simulink model "Eg8_4"  (R2018a)
settings: Solver=VariableStepAuto  StartTime=0.0  StopTime=10000  RelTol=1e-3
settings Model: Creator=wangluo  LastModifiedBy=wangluo

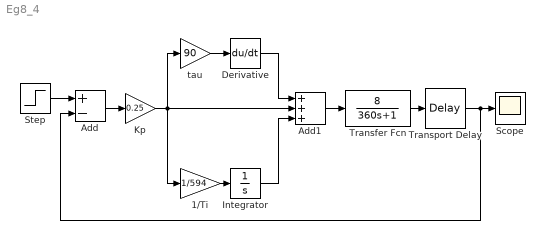
== system Eg8_4 ==
  1/Ti : Gain  Gain=1/594
  Add : Sum  Inputs=+-
  Add1 : Sum  Inputs=+++
  Derivative : Derivative
  Integrator : Integrator
  Kp : Gain  Gain=0.25
  Scope : Scope
  Step : Step  SampleTime=0
  Transfer Fcn : TransferFcn  Numerator=[8]  Denominator=[360 1]
  Transport Delay : TransportDelay  DelayTime=180
  tau : Gain  Gain=90
  wires:
  Step/1 -> Add/1
  Add/1 -> Kp/1
  tau/1 -> Derivative/1
  1/Ti/1 -> Integrator/1
  Kp/1 -> tau/1, 1/Ti/1, Add1/2
  Add1/1 -> Transfer Fcn/1
  Transfer Fcn/1 -> Transport Delay/1
  Transport Delay/1 -> Add/2, Scope/1
  Derivative/1 -> Add1/1
  Integrator/1 -> Add1/3
